simulink library "optiTruck_lib"  (R2016b)
settings: Solver=VariableStepAuto  StartTime=0.0  StopTime=10.0  RelTol=1e-3  EnableMultiTasking=on
libraries: simulink x4, optiTruck_lib x2, simulink_extras x2
settings Model: Creator=tbaumgar  LastModifiedBy=m01wolf
settings DataIOCC: LimitDataPoints=on
settings OptimizationCC: LifeSpan=inf
settings DebuggingCC: AllowSymbolicDim=off  SFUnexpectedBacktrackingDiag=warning  SFNoUnconditionalDefaultTransitionDiag=warning  SFExecutionAtInitializationDiag=none
settings ModelReferenceCC: PropagateSignalLabelsOutOfModel=off
settings GRTTargetCC: TargetLangStandard=C89/C90 (ANSI)
settings ConfigComp: CovMetricSettings=dw  CovHtmlReporting=on  CovSaveCumulativeToWorkspaceVar=on  CovSaveSingleToWorkspaceVar=on  CovExternalEMLEnable=off

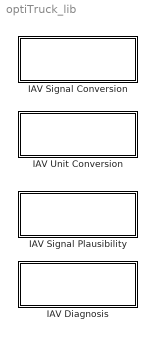
== system optiTruck_lib ==
  IAV Diagnosis : Subsystem
      mask Display: color('white'); text(0.1,0.5,'IAV Diagnosis')
  IAV Signal Conversion : Subsystem
      mask Display: color('white'); text(0.1,0.5,'IAV Signal Conversion')
  IAV Signal Plausibility : Subsystem
      mask Display: color('white'); text(0.1,0.5,'IAV Signal Plausibility')
  IAV Unit Conversion : Subsystem
      mask Display: color('white'); text(0.1,0.5,'IAV Unit Conversion')

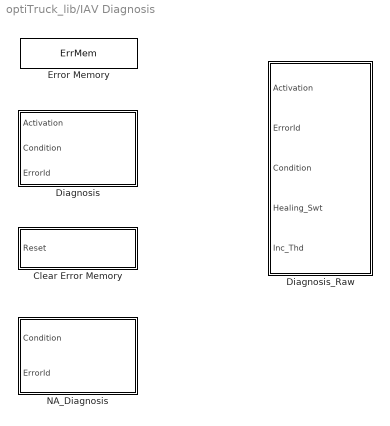
== system optiTruck_lib/IAV Diagnosis ==
  Clear Error Memory : Subsystem
      mask Display: color('white'); port_label('input',1,'Reset')
  Diagnosis : Subsystem  mask{Diag_ErrSetIncThd_Value=255, Diag_HealingActvd_Swt=off, Diag_ErrMem_Size=4}
      mask prompts: Diag_ErrSetIncThd_Value "Incident counter threshold"; Diag_HealingActvd_Swt "Error healing"; Diag_ErrMem_Size "Error Memory Size (bytes)"
      mask Display:
      | color('white'); port_label('input',1,'Activation')
      | color('white'); port_label('input',2,'Condition')
      | color('white'); port_label('input',3,'ErrorID')
  Diagnosis_Raw : Subsystem
  Error Memory : DataStoreMemory  DataStoreName=ErrMem  ReadBeforeWriteMsg=warning  WriteAfterWriteMsg=warning  WriteAfterReadMsg=warning  InitialValue=zeros(1,4,'uint32')  ShowAdditionalParam=off  OutDataTypeStr=uint32
  NA_Diagnosis : Subsystem  mask{Diag_ErrSetIncThd_Value=255, Diag_HealingActvd_Swt=off, Diag_ErrMem_Size=4}
      mask prompts: Diag_ErrSetIncThd_Value "Incident counter threshold"; Diag_HealingActvd_Swt "Error healing"; Diag_ErrMem_Size "Error Memory Size (bytes)"
      mask Display:
      | color('white'); port_label('input',1,'Condition')
      | color('white'); port_label('input',2,'ErrorID')

== system optiTruck_lib/IAV Signal Conversion ==
  Signal Conversion : Subsystem  mask{OutDataTypeStr=Inherit: Inherit via back propagation, OutPortSampleTime=-1}
      mask prompts: OutDataTypeStr "Simulink:blkprm_prompts:OUTPUT_UNIFIEDDATATYPE"; OutPortSampleTime "Simulink:blkprm_prompts:RateTransOutportTs"
      mask TypeOptions OutDataTypeStr: Data Type Conversion/OutDataTypeStr
      mask TypeOptions OutPortSampleTime: Rate Transition/OutPortSampleTime
      mask Display:
      | text(0.1,0.3, ['Type: ' OutDataTypeStr])
      | text(0.1,0.8, ['Sampling [s]: ' num2str(OutPortSampleTime)])

== system optiTruck_lib/IAV Signal Plausibility ==
  Input Signal Check : Subsystem  mask{Inp_Check_Mod_Id=3, Inp_Check_Mod_Str=High limit hysteresis check}
      mask prompts: Inp_Check_Mod_Id "ModeID"; Inp_Check_Mod_Str "Mode"
      mask init:
      | %set_param(gcb, 'Inp_Check_Mod_Id', '0');
      | %set_param(gcb, 'Inp_Check_Mod_Str', 'Range check');
      mask TypeOptions Inp_Check_Mod_Id: Mode/Value
      mask TypeOptions Inp_Check_Mod_Str: High limit check | Low limit check | Range check | High limit hysteresis check | Low limit hysteresis check
      mask Callback Inp_Check_Mod_Str:
      | mode = get_param(gcb, 'Inp_Check_Mod_Str');
      | 
      | mask_obj = get_param(gcb, 'MaskObject');
      | mode_desc_obj = mask_obj.getDialogControl('Inp_Check_Mod_Desc');
      | 
      | switch mode
      |     case 'High limit check'
      |         set_param(gcb, 'Inp_Check_Mod_Id', '0');
      |         mode_desc_obj.Prompt = 'Error flag is set if Signal > Thd_Hi.';
      |     case 'Low limit check'
      |         set_param(gcb, 'Inp_Check_Mod_Id', '1');
      |         mode_desc_obj.Prompt = 'Error flag is set if Signal < Thd_Lo.';
      |     case 'Range check'
      |         set_param(gcb, 'Inp_Check_Mod_Id', '2');
      |         mode_desc_obj.Prompt = 'Error flag is set if Signal > Thd_Hi or Signal < Thd_Lo.';
      |     case 'High limit hysteresis check'
      |         set_param(gcb, 'Inp_Check_Mod_Id', '3');
      |         mode_desc_obj.Prompt = 'Error flag is set when Signal > Thd_Hi and unset when Signal < Thd_Lo.';
      |     case 'Low limit hysteresis check'
      |         set_param(gcb, 'Inp_Check_Mod_Id', '4');
      |         mode_desc_obj.Prompt = 'Error flag is set when Signal < Thd_Lo and unset when Signal > Thd_Hi.';
      | end
      | 
      | clear mode_desc_obj;
      | clear mask_obj;
      | clear mode;
      mask DialogControl DescGroupVar Prompt: Input Signal Check
      mask DialogControl Inp_Check_Mod_Desc Prompt: Error flag is set when Signal > Thd_Hi and unset when Signal < Thd_Lo.
      mask Display:
      | color('white')
      | port_label('input',1,'Signal')
      | port_label('input',2,'Thd_Hi')
      | port_label('input',3,'Thd_Lo')
      | port_label('output',1,'ErrFlg')

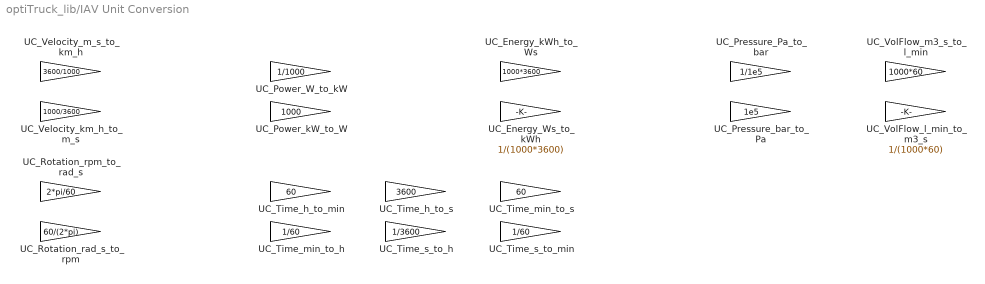
== system optiTruck_lib/IAV Unit Conversion ==
  UC_Energy_Ws_to_kWh : Gain  Gain=1/(1000*3600)
      mask Display:
      | color('white'); port_label('input',1,'Ws')
      | color('white'); port_label('output',1,'kWh')
  UC_Energy_kWh_to_Ws : Gain  Gain=1000*3600
      mask Display:
      | color('white'); port_label('input',1,'kWh')
      | color('white'); port_label('output',1,'Ws')
  UC_Power_W_to_kW : Gain  Gain=1/1000
      mask Display:
      | color('white'); port_label('input',1,'W')
      | color('white'); port_label('output',1,'kW')
  UC_Power_kW_to_W : Gain  Gain=1000
      mask Display:
      | color('white'); port_label('input',1,'kW')
      | color('white'); port_label('output',1,'W')
  UC_Pressure_Pa_to_bar : Gain  Gain=1/1e5
      mask Display:
      | color('white'); port_label('input',1,'Pa')
      | color('white'); port_label('output',1,'bar')
  UC_Pressure_bar_to_Pa : Gain  Gain=1e5
      mask Display:
      | color('white'); port_label('input',1,'bar')
      | color('white'); port_label('output',1,'Pa')
  UC_Rotation_rad_s_to_rpm : Gain  Gain=60/(2*pi)
      mask Display:
      | color('white'); port_label('input',1,'rad/s')
      | color('white'); port_label('output',1,'rpm')
  UC_Rotation_rpm_to_rad_s : Gain  Gain=2*pi/60
      mask Display:
      | color('white'); port_label('input',1,'rpm')
      | color('white'); port_label('output',1,'rad/s')
  UC_Time_h_to_min : Gain  Gain=60
      mask Display:
      | color('white'); port_label('input',1,'h')
      | color('white'); port_label('output',1,'min')
  UC_Time_h_to_s : Gain  Gain=3600
      mask Display:
      | color('white'); port_label('input',1,'h')
      | color('white'); port_label('output',1,'s')
  UC_Time_min_to_h : Gain  Gain=1/60
      mask Display:
      | color('white'); port_label('input',1,'min')
      | color('white'); port_label('output',1,'h')
  UC_Time_min_to_s : Gain  Gain=60
      mask Display:
      | color('white'); port_label('input',1,'min')
      | color('white'); port_label('output',1,'s')
  UC_Time_s_to_h : Gain  Gain=1/3600
      mask Display:
      | color('white'); port_label('input',1,'s')
      | color('white'); port_label('output',1,'h')
  UC_Time_s_to_min : Gain  Gain=1/60
      mask Display:
      | color('white'); port_label('input',1,'s')
      | color('white'); port_label('output',1,'min')
  UC_Velocity_km_h_to_m_s : Gain  Gain=1000/3600
      mask Display:
      | color('white'); port_label('input',1,'km/h')
      | color('white'); port_label('output',1,'m/s')
  UC_Velocity_m_s_to_km_h : Gain  Gain=3600/1000
      mask Display:
      | color('white'); port_label('input',1,'m/s')
      | color('white'); port_label('output',1,'km/h')
  UC_VolFlow_l_min_to_m3_s : Gain  Gain=1/(1000*60)
      mask Display:
      | color('white'); port_label('input',1,'l/min')
      | color('white'); port_label('output',1,'m³/s')
  UC_VolFlow_m3_s_to_l_min : Gain  Gain=1000*60
      mask Display:
      | color('white'); port_label('input',1,'m³/s')
      | color('white'); port_label('output',1,'l/min')

== system optiTruck_lib/IAV Diagnosis/Clear Error Memory ==
  Reset : Inport  OutDataTypeStr=boolean
  Set ErrMem to 0 (each Byte) : Subsystem
  wires:
  Reset/1 -> Set ErrMem to 0 (each Byte)/Enable

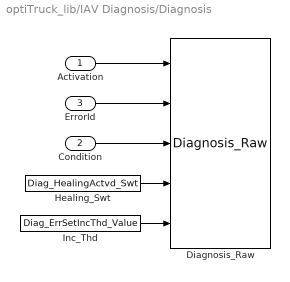
== system optiTruck_lib/IAV Diagnosis/Diagnosis ==
  Activation : Inport  OutMin=0  OutMax=1  OutDataTypeStr=boolean
  Condition : Inport  Port=2  OutDataTypeStr=boolean
  ErrorId : Inport  Port=3
  Diagnosis_Raw : optiTruck_lib/IAV Diagnosis/Diagnosis_Raw
  Healing_Swt : Constant  Value=Diag_HealingActvd_Swt  OutDataTypeStr=boolean
  Inc_Thd : Constant  Value=Diag_ErrSetIncThd_Value  OutDataTypeStr=uint8
  wires:
  Activation/1 -> Diagnosis_Raw/1
  ErrorId/1 -> Diagnosis_Raw/2
  Condition/1 -> Diagnosis_Raw/3
  Healing_Swt/1 -> Diagnosis_Raw/4
  Inc_Thd/1 -> Diagnosis_Raw/5

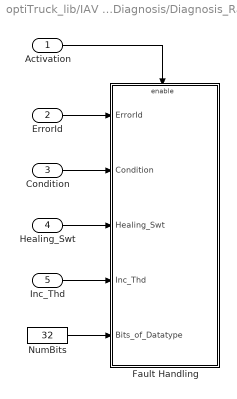
== system optiTruck_lib/IAV Diagnosis/Diagnosis_Raw ==
  Activation : Inport  OutDataTypeStr=boolean
  ErrorId : Inport  Port=2  OutDataTypeStr=uint32
  Condition : Inport  Port=3  OutDataTypeStr=boolean
  Healing_Swt : Inport  Port=4  OutDataTypeStr=boolean
  Inc_Thd : Inport  Port=5  OutDataTypeStr=uint8
  Fault Handling : Subsystem
  NumBits : Constant  Value=32  OutDataTypeStr=uint32
  wires:
  Activation/1 -> Fault Handling/Enable
  Condition/1 -> Fault Handling/2(Condition)
  ErrorId/1 -> Fault Handling/1(ErrorId)
  Healing_Swt/1 -> Fault Handling/3(Healing_Swt)
  Inc_Thd/1 -> Fault Handling/4(Inc_Thd)
  NumBits/1 -> Fault Handling/5(Bits_of_Datatype)

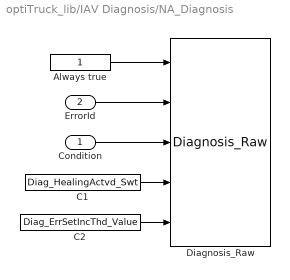
== system optiTruck_lib/IAV Diagnosis/NA_Diagnosis ==
  Condition : Inport  OutDataTypeStr=boolean
  ErrorId : Inport  Port=2
  Always true : Constant  OutDataTypeStr=boolean
  C1 : Constant  Value=Diag_HealingActvd_Swt  OutDataTypeStr=boolean
  C2 : Constant  Value=Diag_ErrSetIncThd_Value  OutDataTypeStr=uint8
  Diagnosis_Raw : optiTruck_lib/IAV Diagnosis/Diagnosis_Raw
  wires:
  C2/1 -> Diagnosis_Raw/5
  C1/1 -> Diagnosis_Raw/4
  Condition/1 -> Diagnosis_Raw/3
  ErrorId/1 -> Diagnosis_Raw/2
  Always true/1 -> Diagnosis_Raw/1

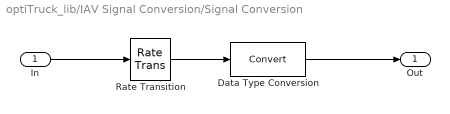
== system optiTruck_lib/IAV Signal Conversion/Signal Conversion ==
  In : Inport
  Data Type Conversion : DataTypeConversion
  Rate Transition : RateTransition  OutPortSampleTime=OutPortSampleTime
  Out : Outport
  wires:
  Rate Transition/1 -> Data Type Conversion/1
  Data Type Conversion/1 -> Out/1
  In/1 -> Rate Transition/1

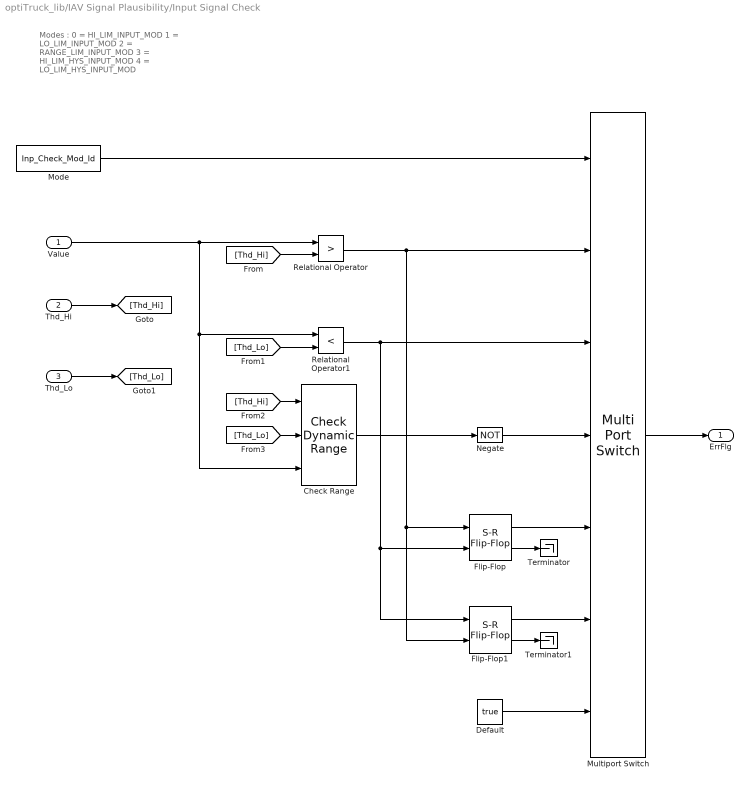
== system optiTruck_lib/IAV Signal Plausibility/Input Signal Check ==
  note: Modes :
      | 0 = HI_LIM_INPUT_MOD
      | 1 = LO_LIM_INPUT_MOD
      | 2 = RANGE_LIM_INPUT_MOD
      | 3 = HI_LIM_HYS_INPUT_MOD
      | 4 = LO_LIM_HYS_INPUT_MOD
  Value : Inport
  Thd_Hi : Inport  Port=2
  Thd_Lo : Inport  Port=3
  Check Range : simulink/Model Verification/Check  Dynamic Range  Description=min < sig < max  enabled=on  stopWhenAssertionFail=off  export=on  icon=text
  Default : Constant  Value=true  OutDataTypeStr=boolean
  Flip-Flop : simulink_extras/Flip Flops/S-R Flip-Flop  initial_condition=0
  Flip-Flop1 : simulink_extras/Flip Flops/S-R Flip-Flop  initial_condition=0
  Mode : Constant  Value=Inp_Check_Mod_Id
  Multiport Switch : MultiPortSwitch  DataPortOrder=Zero-based contiguous  Inputs=6  DataPortIndices={'X',2,3}  DiagnosticForDefault=Warning
  Negate : Logic  Operator=NOT  Inputs=1  AllPortsSameDT=off  OutDataTypeStr=boolean
  Relational Operator : RelationalOperator  Operator=>  OutDataTypeStr=boolean  RndMeth=Simplest
  Relational Operator1 : RelationalOperator  Operator=<  OutDataTypeStr=boolean  RndMeth=Simplest
  Terminator : Terminator
  Terminator1 : Terminator
  ErrFlg : Outport  OutDataTypeStr=boolean
  wires:
  Mode/1 -> Multiport Switch/1
  Relational Operator/1 -> Flip-Flop/1, Flip-Flop1/2, Multiport Switch/2
  Thd_Hi/1 -> [Thd_Hi]
  [Thd_Hi] -> Relational Operator/2
  Value/1 -> Check Range/3, Relational Operator1/1, Relational Operator/1
  [Thd_Lo] -> Relational Operator1/2
  Thd_Lo/1 -> [Thd_Lo]
  Check Range/1 -> Negate/1
  [Thd_Hi] -> Check Range/1
  [Thd_Lo] -> Check Range/2
  Relational Operator1/1 -> Flip-Flop/2, Flip-Flop1/1, Multiport Switch/3
  Default/1 -> Multiport Switch/7
  Multiport Switch/1 -> ErrFlg/1
  Negate/1 -> Multiport Switch/4
  Flip-Flop/1 -> Multiport Switch/5
  Flip-Flop1/1 -> Multiport Switch/6
  Flip-Flop/2 -> Terminator/1
  Flip-Flop1/2 -> Terminator1/1

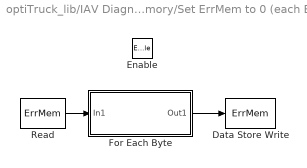
== system optiTruck_lib/IAV Diagnosis/Clear Error Memory/Set ErrMem to 0 (each Byte) ==
  Enable : EnablePort
  Data Store Write : DataStoreWrite  DataStoreName=ErrMem
  For Each Byte : Subsystem  TreatAsAtomicUnit=on
  Read : DataStoreRead  DataStoreName=ErrMem
  wires:
  Read/1 -> For Each Byte/1(In1)
  For Each Byte/1(Out1) -> Data Store Write/1

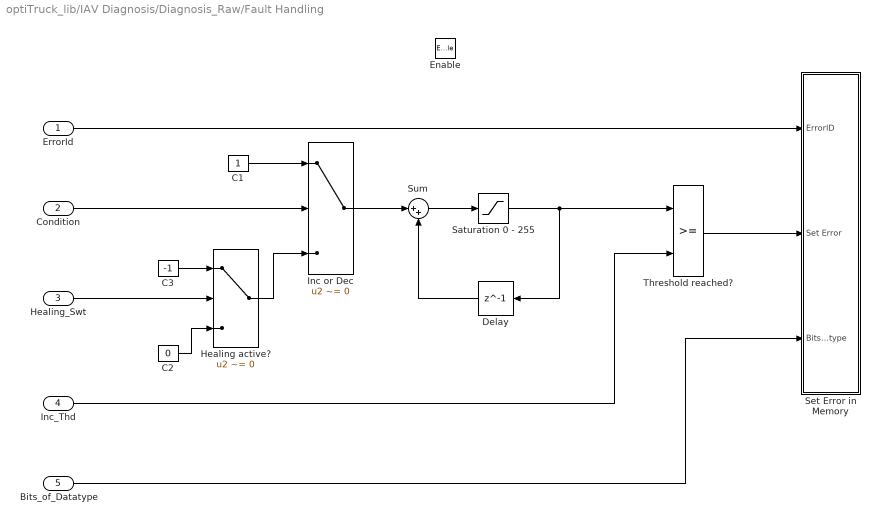
== system optiTruck_lib/IAV Diagnosis/Diagnosis_Raw/Fault Handling ==
  ErrorId : Inport
  Condition : Inport  Port=2  OutDataTypeStr=boolean
  Healing_Swt : Inport  Port=3  OutDataTypeStr=boolean
  Inc_Thd : Inport  Port=4  OutDataTypeStr=uint8
  Bits_of_Datatype : Inport  Port=5  OutDataTypeStr=uint32
  Enable : EnablePort
  C1 : Constant  OutDataTypeStr=int8
  C2 : Constant  Value=0  OutDataTypeStr=int8
  C3 : Constant  Value=-1  OutDataTypeStr=int8
  Delay : Delay  DelayLength=1
  Healing active? : Switch  Criteria=u2 ~= 0
  Inc or Dec : Switch  Criteria=u2 ~= 0
  Saturation 0 - 255 : Saturate  UpperLimit=255  LowerLimit=0  OutDataTypeStr=uint8
  Set Error in Memory : Subsystem
  Sum : Sum  Inputs=|++  OutDataTypeStr=int8
  Threshold reached? : RelationalOperator  OutDataTypeStr=boolean  RndMeth=Simplest
  wires:
  C1/1 -> Inc or Dec/1
  Sum/1 -> Saturation 0 - 255/1
  Inc or Dec/1 -> Sum/1
  ErrorId/1 -> Set Error in Memory/1(ErrorID)
  Saturation 0 - 255/1 -> Threshold reached?/1, Delay/1
  Threshold reached?/1 -> Set Error in Memory/2(Set Error)
  Delay/1 -> Sum/2
  Condition/1 -> Inc or Dec/2
  C2/1 -> Healing active?/3
  Healing active?/1 -> Inc or Dec/3
  C3/1 -> Healing active?/1
  Healing_Swt/1 -> Healing active?/2
  Inc_Thd/1 -> Threshold reached?/2
  Bits_of_Datatype/1 -> Set Error in Memory/3(Bits_of_Datatype)

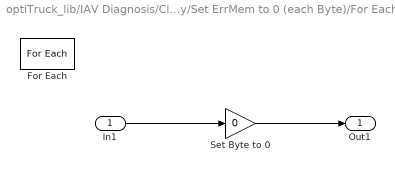
== system optiTruck_lib/IAV Diagnosis/Clear Error Memory/Set ErrMem to 0 (each Byte)/For Each Byte ==
  In1 : Inport  Partition=on  PartitionDimension=1  PartitionWidth=1
  For Each : ForEach  DisableCoverage=on  IndexMode=One-based
  Set Byte to 0 : Gain  Gain=0  OutDataTypeStr=uint8
  Out1 : Outport  ConcatenationDimension=1
  wires:
  In1/1 -> Set Byte to 0/1
  Set Byte to 0/1 -> Out1/1

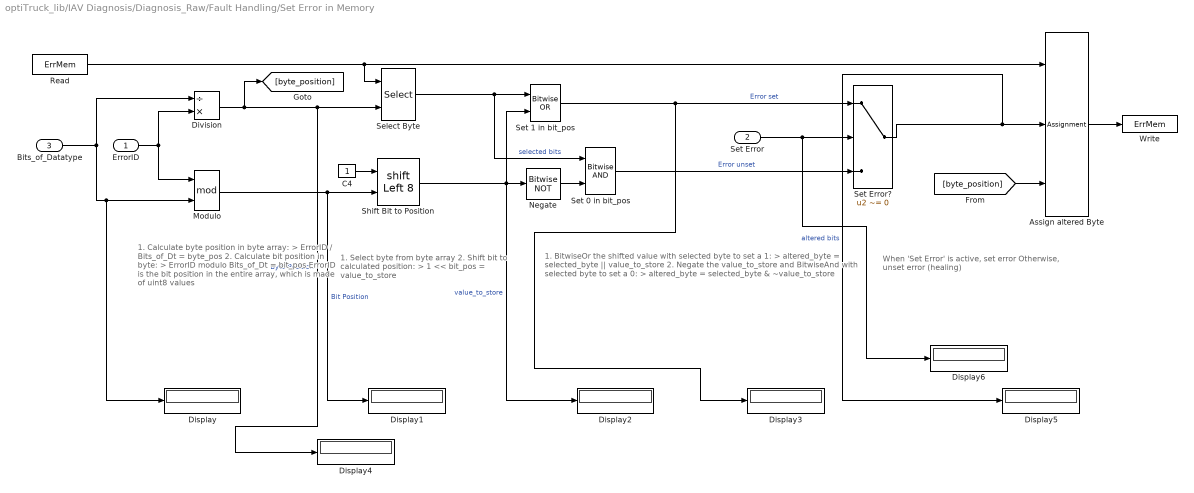
== system optiTruck_lib/IAV Diagnosis/Diagnosis_Raw/Fault Handling/Set Error in Memory ==
  note: 1. Calculate byte position in byte array:
      | > ErrorID / Bits_of_Dt = byte_pos
      |
      | 2. Calculate bit position in byte:
      | > ErrorID modulo Bits_of_Dt = bit_pos
      |
      | ErrorID is the bit position in the entire array, which is made of uint8 values
  note: 1. Select byte from byte array
      |
      | 2. Shift bit to calculated position:
      | > 1 << bit_pos = value_to_store
  note: 1. BitwiseOr the shifted value with selected byte to set a 1:
      | > altered_byte = selected_byte || value_to_store
      |
      | 2. Negate the value_to_store and BitwiseAnd with selected byte to set a 0:
      | > altered_byte = selected_byte & ~value_to_store
  note: When 'Set Error' is active, set error
      |
      | Otherwise, unset error (healing)
  ErrorID : Inport  OutDataTypeStr=uint32
  Set Error : Inport  Port=2
  Bits_of_Datatype : Inport  Port=3  OutDataTypeStr=uint32
  Assign altered Byte : Assignment  IndexMode=Zero-based  DiagnosticForDimensions=Warning  IndexOptions=Index vector (port)  Indices=1  OutputSizes=1
  C4 : Constant  OutDataTypeStr=uint32
  Display{,1..6} (7 alike) : Display
  Division : Product  Inputs=/*  OutDataTypeStr=uint32
  Modulo : Math  Operator=mod  OutputSignalType=real  SaturateOnIntegerOverflow=on
  Negate : simulink/Logic and Bit Operations/Bitwise Operator  logicop=NOT  UseBitMask=off  BitMask=bin2dec('11011001')  BitMaskRealWorld=Real World Value
  Read : DataStoreRead  DataStoreName=ErrMem
  Select Byte : Selector  IndexMode=Zero-based  InputPortWidth=Diag_ErrMem_Size  IndexOptions=Index vector (port)  Indices=[1 3]  OutputSizes=1
  Set 0 in bit_pos : simulink/Logic and Bit Operations/Bitwise Operator  logicop=AND  UseBitMask=off  NumInputPorts=2  BitMask=bin2dec('11011001')  BitMaskRealWorld=Real World Value
  Set 1 in bit_pos : simulink/Logic and Bit Operations/Bitwise Operator  logicop=OR  UseBitMask=off  NumInputPorts=2  BitMask=bin2dec('11011001')  BitMaskRealWorld=Real World Value
  Set Error? : Switch  Criteria=u2 ~= 0  OutDataTypeStr=uint32
  Shift Bit to Position : ArithShift  BitShiftNumberSource=Input port  BitShiftNumber=8  BitShiftDirection=Left
      settings: InputPortMap=u0,p1
  Write : DataStoreWrite  DataStoreName=ErrMem
  wires:
  Assign altered Byte/1 -> Write/1
  Modulo/1 -> Display1/1, Shift Bit to Position/2  "Bit Position"
  ErrorID/1 -> Modulo/1, Division/2
  C4/1 -> Shift Bit to Position/1
  Set 0 in bit_pos/1 -> Set Error?/3  "Error unset"
  Select Byte/1 -> Set 1 in bit_pos/1, Set 0 in bit_pos/1  "selected bits"
  Shift Bit to Position/1 -> Display2/1, Set 1 in bit_pos/2, Negate/1  "value_to_store"
  Read/1 -> Select Byte/1, Assign altered Byte/1
  Division/1 -> Display4/1, Select Byte/2, [byte_position]  "Byte Position"
  [byte_position] -> Assign altered Byte/3
  Bits_of_Datatype/1 -> Display/1, Modulo/2, Division/1
  Set Error/1 -> Display6/1, Set Error?/2
  Negate/1 -> Set 0 in bit_pos/2
  Set 1 in bit_pos/1 -> Display3/1, Set Error?/1  "Error set"
  Set Error?/1 -> Display5/1, Assign altered Byte/2  "altered bits"
